simulink model "penduloInvNoLinealRealimentadoCorre"  (Simulink 7.3)
settings: Solver=ode45  StartTime=0.0  StopTime=10  RelTol=1e-3
values from neighbouring files (symbols this model uses):
  K = lqr(A,B,Q,R)    [LQR.m]    (also in bestQ.m = setK_lqr(Q_i); graficosPenduloReal.m = setK_lqr(Q_optimo))
libraries: simulink x10
settings Model: Creator=Daniel  LastModifiedBy=Daniel

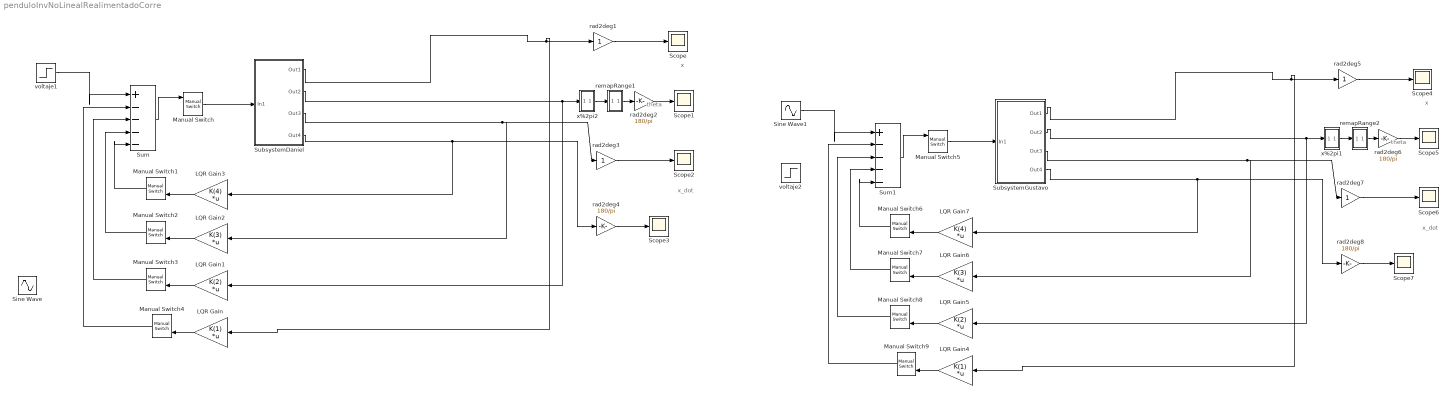
== system penduloInvNoLinealRealimentadoCorre ==
  note: x
  note: theta
  note: x_dot
  note: x
  note: theta
  note: x_dot
  LQR Gain : Gain  Gain=K(1)  Multiplication=Matrix(K*u)  SampleTime=0.1  SaturateOnIntegerOverflow=on  OutDataTypeStr=Inherit: Same as input  ParamDataTypeStr=Inherit: Same as input
  LQR Gain1 : Gain  Gain=K(2)  Multiplication=Matrix(K*u)  SampleTime=0.1  SaturateOnIntegerOverflow=on  OutDataTypeStr=Inherit: Same as input  ParamDataTypeStr=Inherit: Same as input
  LQR Gain2 : Gain  Gain=K(3)  Multiplication=Matrix(K*u)  SampleTime=0.1  SaturateOnIntegerOverflow=on  OutDataTypeStr=Inherit: Same as input  ParamDataTypeStr=Inherit: Same as input
  LQR Gain3 : Gain  Gain=K(4)  Multiplication=Matrix(K*u)  SampleTime=0.1  SaturateOnIntegerOverflow=on  OutDataTypeStr=Inherit: Same as input  ParamDataTypeStr=Inherit: Same as input
  LQR Gain4 : Gain  Gain=K(1)  Multiplication=Matrix(K*u)  SampleTime=0.1  SaturateOnIntegerOverflow=on  OutDataTypeStr=Inherit: Same as input  ParamDataTypeStr=Inherit: Same as input
  LQR Gain5 : Gain  Gain=K(2)  Multiplication=Matrix(K*u)  SampleTime=0.1  SaturateOnIntegerOverflow=on  OutDataTypeStr=Inherit: Same as input  ParamDataTypeStr=Inherit: Same as input
  LQR Gain6 : Gain  Gain=K(3)  Multiplication=Matrix(K*u)  SampleTime=0.1  SaturateOnIntegerOverflow=on  OutDataTypeStr=Inherit: Same as input  ParamDataTypeStr=Inherit: Same as input
  LQR Gain7 : Gain  Gain=K(4)  Multiplication=Matrix(K*u)  SampleTime=0.1  SaturateOnIntegerOverflow=on  OutDataTypeStr=Inherit: Same as input  ParamDataTypeStr=Inherit: Same as input
  Manual Switch : simulink/Signal Routing/Manual Switch  SystemSampleTime=-1  sw=1  action=0  varsize=off
  Manual Switch{1..4,6..9} (8 alike) : simulink/Signal Routing/Manual Switch  SystemSampleTime=-1  sw=0  action=0  varsize=off
  Manual Switch5 : simulink/Signal Routing/Manual Switch  SystemSampleTime=-1  sw=1  action=0  varsize=off
  Scope{,1..7} (8 alike) : Scope
      Scope1 settings: SaveName=ScopeData2
      Scope2 settings: SaveName=ScopeData3
      Scope3 settings: SaveName=ScopeData4
      Scope4 settings: SaveName=ScopeData6
      Scope5 settings: SaveName=ScopeData7
      Scope6 settings: SaveName=ScopeData8
      Scope7 settings: SaveName=ScopeData9
  Sine Wave : Sin  Amplitude=2  Bias=0  Frequency=10  Phase=0  Samples=10  SampleTime=0.1  Offset=0
  Sine Wave1 : Sin  Amplitude=2  Bias=0  Frequency=10  Phase=0  Samples=10  SampleTime=0.1  Offset=0
  SubsystemDaniel : Subsystem
  SubsystemGustavo : Subsystem
  Sum : Sum  Inputs=|+----  SampleTime=0.1
  Sum1 : Sum  Inputs=|+----  SampleTime=0.1
  rad2deg{1,3,5,7} (4 alike) : Gain  SaturateOnIntegerOverflow=on  OutDataTypeStr=Inherit: Same as input  ParamDataTypeStr=Inherit: Same as input
  rad2deg{2,4,6,8} (4 alike) : Gain  Gain=180/pi  SaturateOnIntegerOverflow=on  OutDataTypeStr=Inherit: Same as input  ParamDataTypeStr=Inherit: Same as input
  remapRange1 : Stateflow chart  TreatAsAtomicUnit=on
  remapRange2 : Stateflow chart  TreatAsAtomicUnit=on
  voltaje1 : Step  Time=0  After=5  SampleTime=0
  voltaje2 : Step  Time=0  After=5  SampleTime=0
  x%2pi1 : Stateflow chart  TreatAsAtomicUnit=on
  x%2pi2 : Stateflow chart  TreatAsAtomicUnit=on
  wires:
  rad2deg4/1 -> Scope3/1
  rad2deg3/1 -> Scope2/1
  SubsystemDaniel/3(Out3) -> LQR Gain2/1, rad2deg3/1
  rad2deg1/1 -> Scope/1
  SubsystemDaniel/1(Out1) -> rad2deg1/1, LQR Gain/1
  SubsystemDaniel/2(Out2) -> LQR Gain1/1, x%2pi2/1(u)
  LQR Gain3/1 -> Manual Switch1/2
  LQR Gain2/1 -> Manual Switch2/2
  LQR Gain1/1 -> Manual Switch3/2
  Manual Switch/1 -> SubsystemDaniel/1(In1)
  SubsystemDaniel/4(Out4) -> rad2deg4/1, LQR Gain3/1
  Sum/1 -> Manual Switch/1
  rad2deg2/1 -> Scope1/1
  LQR Gain/1 -> Manual Switch4/2
  x%2pi2/1(y) -> remapRange1/1(value)
  remapRange1/1(y) -> rad2deg2/1
  Manual Switch1/1 -> Sum/5
  Manual Switch2/1 -> Sum/4
  Manual Switch3/1 -> Sum/3
  Manual Switch4/1 -> Sum/2
  voltaje1/1 -> Sum/1
  rad2deg8/1 -> Scope7/1
  rad2deg7/1 -> Scope6/1
  SubsystemGustavo/3(Out3) -> LQR Gain6/1, rad2deg7/1
  rad2deg5/1 -> Scope4/1
  SubsystemGustavo/1(Out1) -> rad2deg5/1, LQR Gain4/1
  SubsystemGustavo/2(Out2) -> LQR Gain5/1, x%2pi1/1(u)
  LQR Gain7/1 -> Manual Switch6/2
  LQR Gain6/1 -> Manual Switch7/2
  LQR Gain5/1 -> Manual Switch8/2
  Manual Switch5/1 -> SubsystemGustavo/1(In1)
  SubsystemGustavo/4(Out4) -> rad2deg8/1, LQR Gain7/1
  Sum1/1 -> Manual Switch5/1
  rad2deg6/1 -> Scope5/1
  LQR Gain4/1 -> Manual Switch9/2
  x%2pi1/1(y) -> remapRange2/1(value)
  remapRange2/1(y) -> rad2deg6/1
  Manual Switch6/1 -> Sum1/5
  Manual Switch7/1 -> Sum1/4
  Manual Switch8/1 -> Sum1/3
  Manual Switch9/1 -> Sum1/2
  Sine Wave1/1 -> Sum1/1

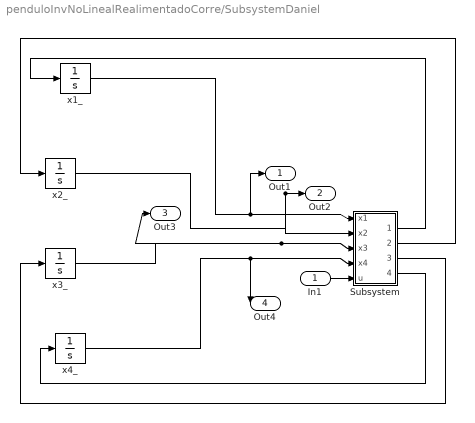
== system penduloInvNoLinealRealimentadoCorre/SubsystemDaniel ==
  In1 : Inport
  Subsystem : Subsystem
  x1_ : Integrator  LimitOutput=on  UpperSaturationLimit=100  LowerSaturationLimit=-100
  x2_ : Integrator  InitialCondition=190*pi/180  UpperSaturationLimit=2*pi  LowerSaturationLimit=0
  x3_ : Integrator  LimitOutput=on  UpperSaturationLimit=100  LowerSaturationLimit=-100
  x4_ : Integrator  LimitOutput=on  UpperSaturationLimit=100  LowerSaturationLimit=-100
  Out1 : Outport
  Out2 : Outport  Port=2
  Out3 : Outport  Port=3
  Out4 : Outport  Port=4
  wires:
  x1_/1 -> Subsystem/1(x1), Out1/1
  Subsystem/1(phi1) -> x1_/1
  Subsystem/2(phi2) -> x2_/1
  Subsystem/3(phi3) -> x3_/1
  Subsystem/4(phi4) -> x4_/1
  x2_/1 -> Subsystem/2(x2), Out2/1
  x3_/1 -> Subsystem/3(x3), Out3/1
  x4_/1 -> Subsystem/4(x4), Out4/1
  In1/1 -> Subsystem/5(u)

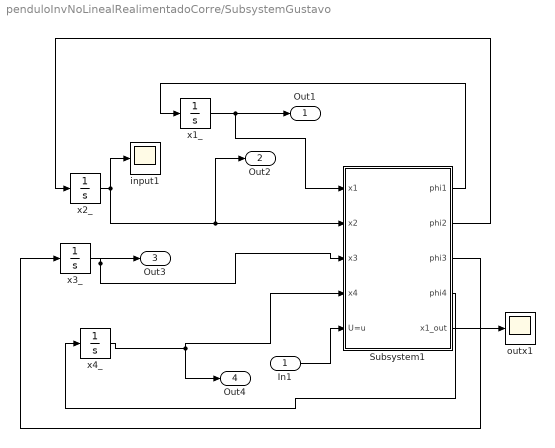
== system penduloInvNoLinealRealimentadoCorre/SubsystemGustavo ==
  In1 : Inport
  Subsystem1 : Subsystem
  input1 : Scope
      settings: SaveName=ScopeData5
  outx1 : Scope
  x1_ : Integrator  LimitOutput=on  UpperSaturationLimit=6  LowerSaturationLimit=-6
  x2_ : Integrator  InitialCondition=180*pi/180  UpperSaturationLimit=2*pi  LowerSaturationLimit=0
  x3_ : Integrator  LimitOutput=on  UpperSaturationLimit=5  LowerSaturationLimit=-5
  x4_ : Integrator  LimitOutput=on  UpperSaturationLimit=5  LowerSaturationLimit=-5
  Out1 : Outport
  Out2 : Outport  Port=2
  Out3 : Outport  Port=3
  Out4 : Outport  Port=4
  wires:
  Subsystem1/2(phi2) -> x2_/1
  Subsystem1/3(phi3) -> x3_/1
  Subsystem1/4(phi4) -> x4_/1
  x4_/1 -> Out4/1, Subsystem1/4(x4)
  Subsystem1/5(x1_out) -> outx1/1
  In1/1 -> Subsystem1/5(U=u)
  x3_/1 -> Out3/1, Subsystem1/3(x3)
  Subsystem1/1(phi1) -> x1_/1
  x1_/1 -> Out1/1, Subsystem1/1(x1)
  x2_/1 -> input1/1, Subsystem1/2(x2), Out2/1

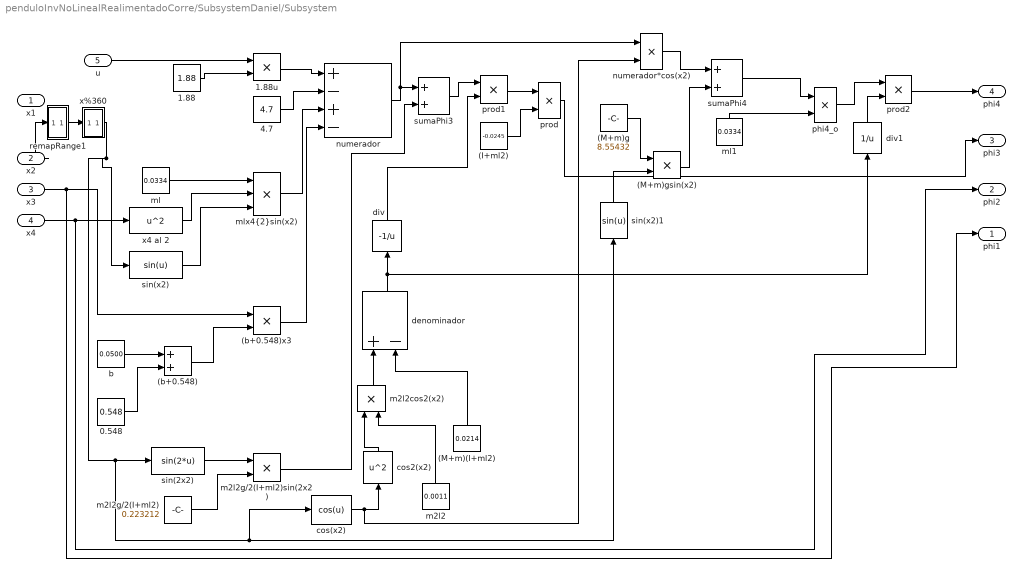
== system penduloInvNoLinealRealimentadoCorre/SubsystemDaniel/Subsystem ==
  x1 : Inport
  x2 : Inport  Port=2
  x3 : Inport  Port=3
  x4 : Inport  Port=4
  u : Inport  Port=5
  (I+ml2) : Constant  Value=-0.0245
  (M+m)(I+ml2) : Constant  Value=0.0214
  (M+m)g : Constant  Value=8.55432
  (M+m)gsin(x2) : Product  RndMeth=Zero
  (b+0.548) : Sum
  (b+0.548)x3 : Product  RndMeth=Zero
  0.548 : Constant  Value=0.548
  1.88 : Constant  Value=1.88
  1.88u : Product  RndMeth=Zero
  4.7 : Constant  Value=4.7
  b : Constant  Value=0.0500
  cos(x2) : Fcn  Expr=cos(u)  SampleTime=0.1
  cos2(x2) : Fcn  Expr=u^2  SampleTime=0.1
  denominador : Sum  Inputs=+-
  div : Fcn  Expr=-1/u  SampleTime=0.1
  div1 : Fcn  Expr=1/u  SampleTime=0.1
  m2l2 : Constant  Value=0.0011
  m2l2cos2(x2) : Product  RndMeth=Zero
  m2l2g/2(I+ml2) : Constant  Value=0.223212
  m2l2g/2(I+ml2)sin(2x2) : Product  RndMeth=Zero
  ml : Constant  Value=0.0334
  ml1 : Constant  Value=0.0334
  "mlx4{2}sin(x2)" : Product  Inputs=3  RndMeth=Zero
  numerador : Sum  Inputs=+-+-
  numerador*cos(x2) : Product  RndMeth=Zero
  phi4_o : Product  RndMeth=Zero
  prod : Product  RndMeth=Zero
  prod1 : Product  RndMeth=Zero
  prod2 : Product  RndMeth=Zero
  remapRange1 : Stateflow chart  TreatAsAtomicUnit=on
  sin(2x2) : Fcn  Expr=sin(2*u)  SampleTime=0.1
  sin(x2) : Fcn  Expr=sin(u)  SampleTime=0.1
  sin(x2)1 : Fcn  Expr=sin(u)  SampleTime=0.1
  sumaPhi3 : Sum
  sumaPhi4 : Sum
  x%360 : Stateflow chart  TreatAsAtomicUnit=on
  x4 al 2 : Fcn  Expr=u^2  SampleTime=0.1
  phi1 : Outport
  phi2 : Outport  Port=2
  phi3 : Outport  Port=3
  phi4 : Outport  Port=4
  wires:
  1.88/1 -> 1.88u/2
  u/1 -> 1.88u/1
  1.88u/1 -> numerador/1
  4.7/1 -> numerador/2
  ml/1 -> "mlx4{2}sin(x2)"/1
  sin(x2)/1 -> "mlx4{2}sin(x2)"/3
  x4 al 2/1 -> "mlx4{2}sin(x2)"/2
  x4/1 -> x4 al 2/1, phi2/1
  "mlx4{2}sin(x2)"/1 -> numerador/3
  (b+0.548)x3/1 -> numerador/4
  x3/1 -> (b+0.548)x3/1, phi1/1
  (b+0.548)/1 -> (b+0.548)x3/2
  b/1 -> (b+0.548)/1
  0.548/1 -> (b+0.548)/2
  sin(2x2)/1 -> m2l2g/2(I+ml2)sin(2x2)/1
  m2l2g/2(I+ml2)/1 -> m2l2g/2(I+ml2)sin(2x2)/2
  m2l2cos2(x2)/1 -> denominador/1
  cos2(x2)/1 -> m2l2cos2(x2)/1
  m2l2/1 -> m2l2cos2(x2)/2
  cos(x2)/1 -> cos2(x2)/1, numerador*cos(x2)/2
  prod1/1 -> prod/1
  (I+ml2)/1 -> prod/2
  ml1/1 -> phi4_o/2
  denominador/1 -> div/1, div1/1
  div/1 -> prod1/2
  x2/1 -> remapRange1/1(value)
  prod/1 -> phi3/1
  sin(x2)1/1 -> (M+m)gsin(x2)/2
  (M+m)g/1 -> (M+m)gsin(x2)/1
  (M+m)(I+ml2)/1 -> denominador/2
  sumaPhi3/1 -> prod1/1
  numerador/1 -> sumaPhi3/1, numerador*cos(x2)/1
  numerador*cos(x2)/1 -> sumaPhi4/1
  (M+m)gsin(x2)/1 -> sumaPhi4/2
  sumaPhi4/1 -> phi4_o/1
  phi4_o/1 -> prod2/1
  div1/1 -> prod2/2
  prod2/1 -> phi4/1
  m2l2g/2(I+ml2)sin(2x2)/1 -> sumaPhi3/2
  remapRange1/1(y) -> x%360/1(u)
  x%360/1(y) -> sin(2x2)/1, cos(x2)/1, sin(x2)1/1, sin(x2)/1

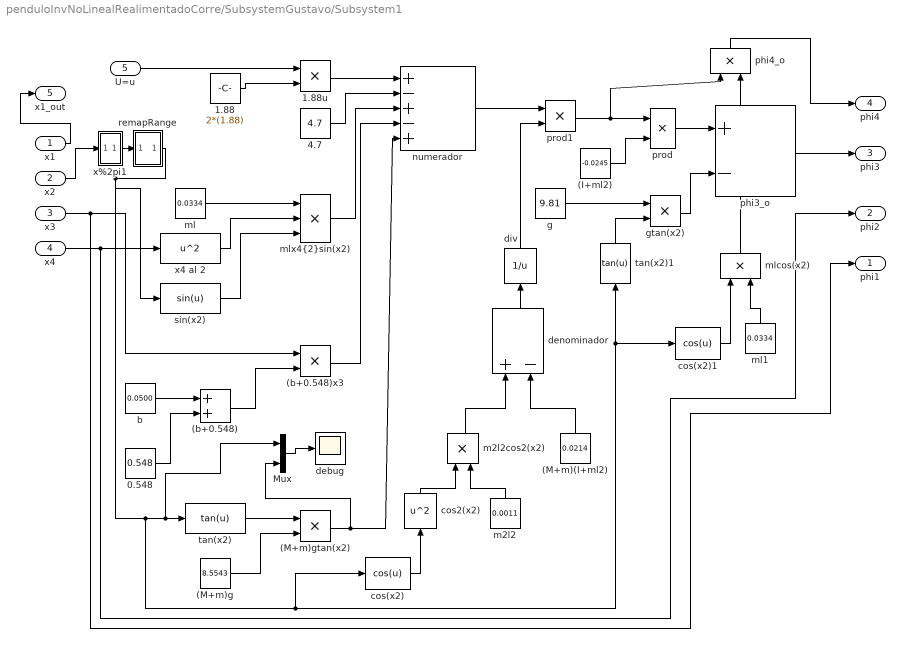
== system penduloInvNoLinealRealimentadoCorre/SubsystemGustavo/Subsystem1 ==
  x1 : Inport
  x2 : Inport  Port=2
  x3 : Inport  Port=3
  x4 : Inport  Port=4
  U=u : Inport  Port=5
  (I+ml2) : Constant  Value=-0.0245
  (M+m)(I+ml2) : Constant  Value=0.0214
  (M+m)g : Constant  Value=8.5543
  (M+m)gtan(x2) : Product  RndMeth=Zero
  (b+0.548) : Sum
  (b+0.548)x3 : Product  RndMeth=Zero
  0.548 : Constant  Value=0.548
  1.88 : Constant  Value=2*(1.88)
  1.88u : Product  RndMeth=Zero
  4.7 : Constant  Value=4.7
  Mux : Mux  Inputs=2
  b : Constant  Value=0.0500
  cos(x2) : Fcn  Expr=cos(u)  SampleTime=0.1
  cos(x2)1 : Fcn  Expr=cos(u)  SampleTime=0.1
  cos2(x2) : Fcn  Expr=u^2  SampleTime=0.1
  debug : Scope
      settings: SaveName=debug
  denominador : Sum  Inputs=+-
  div : Fcn  Expr=1/u  SampleTime=0.1
  g : Constant  Value=9.81
  gtan(x2) : Product  RndMeth=Zero
  m2l2 : Constant  Value=0.0011
  m2l2cos2(x2) : Product  RndMeth=Zero
  ml : Constant  Value=0.0334
  ml1 : Constant  Value=0.0334
  mlcos(x2) : Product  RndMeth=Zero
  "mlx4{2}sin(x2)" : Product  Inputs=3  RndMeth=Zero
  numerador : Sum  Inputs=+-+-+
  phi3_o : Sum  Inputs=+-
  phi4_o : Product  RndMeth=Zero
  prod : Product  RndMeth=Zero
  prod1 : Product  RndMeth=Zero
  remapRange : Stateflow chart  TreatAsAtomicUnit=on
  sin(x2) : Fcn  Expr=sin(u)  SampleTime=0.1
  tan(x2) : Fcn  Expr=tan(u)  SampleTime=0.1
  tan(x2)1 : Fcn  Expr=tan(u)  SampleTime=0.1
  x%2pi1 : Stateflow chart  TreatAsAtomicUnit=on
  x4 al 2 : Fcn  Expr=u^2  SampleTime=0.1
  phi1 : Outport
  phi2 : Outport  Port=2
  phi3 : Outport  Port=3
  phi4 : Outport  Port=4
  x1_out : Outport  Port=5
  wires:
  1.88/1 -> 1.88u/2
  U=u/1 -> 1.88u/1
  1.88u/1 -> numerador/1
  4.7/1 -> numerador/2
  ml/1 -> "mlx4{2}sin(x2)"/1
  sin(x2)/1 -> "mlx4{2}sin(x2)"/3
  x4 al 2/1 -> "mlx4{2}sin(x2)"/2
  x4/1 -> x4 al 2/1, phi2/1
  "mlx4{2}sin(x2)"/1 -> numerador/3
  (b+0.548)x3/1 -> numerador/4
  x3/1 -> phi1/1, (b+0.548)x3/1
  (b+0.548)/1 -> (b+0.548)x3/2
  b/1 -> (b+0.548)/1
  0.548/1 -> (b+0.548)/2
  (M+m)gtan(x2)/1 -> numerador/5, Mux/2
  tan(x2)/1 -> (M+m)gtan(x2)/1
  (M+m)g/1 -> (M+m)gtan(x2)/2
  (M+m)(I+ml2)/1 -> denominador/2
  m2l2cos2(x2)/1 -> denominador/1
  cos2(x2)/1 -> m2l2cos2(x2)/1
  m2l2/1 -> m2l2cos2(x2)/2
  cos(x2)/1 -> cos2(x2)/1
  numerador/1 -> prod1/1
  prod1/1 -> prod/1, phi4_o/1
  (I+ml2)/1 -> prod/2
  prod/1 -> phi3_o/1
  g/1 -> gtan(x2)/1
  tan(x2)1/1 -> gtan(x2)/2
  mlcos(x2)/1 -> phi4_o/2
  ml1/1 -> mlcos(x2)/2
  cos(x2)1/1 -> mlcos(x2)/1
  denominador/1 -> div/1
  div/1 -> prod1/2
  x1/1 -> x1_out/1
  Mux/1 -> debug/1
  x2/1 -> x%2pi1/1(u)
  gtan(x2)/1 -> phi3_o/2
  x%2pi1/1(y) -> remapRange/1(value)
  remapRange/1(y) -> cos(x2)/1, tan(x2)1/1, cos(x2)1/1, tan(x2)/1, Mux/1, sin(x2)/1
  phi4_o/1 -> phi4/1
  phi3_o/1 -> phi3/1

== matlab function SubsystemGustavo/Subsystem1/remapRange ==
  data: value input double; y output double
function y = remapRange(value)
    scaleFactor = pi/180;
    if (value>180*scaleFactor)
        %constants
        fromLow = 181*scaleFactor;
        fromHigh = 360*scaleFactor;
        toLow = -179*scaleFactor;
        toHigh = 0*scaleFactor;
        %calculations
        new_range = toHigh-toLow;
        old_range = fromHigh - fromLow;
        new_value = (new_range/old_range)*(value-fromLow)+toLow;
        y = new_value;
    else
        y = value;
    end
        
end

== matlab function SubsystemGustavo/Subsystem1/x%2pi1 ==
  data: u input double; y output double
function y = fcn(u)
%#codegen

    y = mod(u,2*pi);
end

== matlab function remapRange2 ==
  data: value input double; y output double
function y = remapRange(value)
    scaleFactor = pi/180;
    if (value>180*scaleFactor)
        %constants
        fromLow = 181*scaleFactor;
        fromHigh = 360*scaleFactor;
        toLow = -179*scaleFactor;
        toHigh = 0*scaleFactor;
        %calculations
        new_range = toHigh-toLow;
        old_range = fromHigh - fromLow;
        new_value = (new_range/old_range)*(value-fromLow)+toLow;
        y = new_value;
    else
        y = value;
    end
        
end

== matlab function x%2pi1 ==
  data: u input double; y output double
function y = fcn(u)
%#codegen
    y = mod(u,2*pi);
end

== matlab function remapRange1 ==
  data: value input double; y output double
function y = remapRange(value)
    scaleFactor = pi/180;
    if (value>180*scaleFactor)
        %constants
        fromLow = 181*scaleFactor;
        fromHigh = 360*scaleFactor;
        toLow = -179*scaleFactor;
        toHigh = 0*scaleFactor;
        %calculations
        new_range = toHigh-toLow;
        old_range = fromHigh - fromLow;
        new_value = (new_range/old_range)*(value-fromLow)+toLow;
        y = new_value;
    else
        y = value;
    end
        
end

== matlab function x%2pi2 ==
  data: u input double; y output double
function y = fcn(u)
%#codegen
    y = mod(u,2*pi);
end

== matlab function SubsystemDaniel/Subsystem/remapRange1 ==
  data: value input double; y output double
function y = remapRange(value)
    scaleFactor = pi/180;
    if (value>180*scaleFactor)
        %constants
        fromLow = 181*scaleFactor;
        fromHigh = 360*scaleFactor;
        toLow = -179*scaleFactor;
        toHigh = 0*scaleFactor;
        %calculations
        new_range = toHigh-toLow;
        old_range = fromHigh - fromLow;
        new_value = (new_range/old_range)*(value-fromLow)+toLow;
        y = new_value;
    else
        y = value;
    end
        
end

== matlab function SubsystemDaniel/Subsystem/x%360 ==
  data: u input double; y output double
function y = fcn(u)
%#codegen

    y = mod(u,2*pi);
end
